simulink model "pasaBajoSimuLink"  (R2014b)
settings: Solver=ode45  StartTime=0.0  StopTime=10.0  RelTol=1e-3
settings Model: Creator=Chehin  LastModifiedBy=Chehin

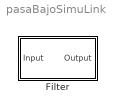
== system pasaBajoSimuLink ==
  Filter : Subsystem  Tag=FilterWizardSubSystem
      settings: ErrorFcn=dspFilterRealizedInBasicElemsAlgLoopErrFcnCallback

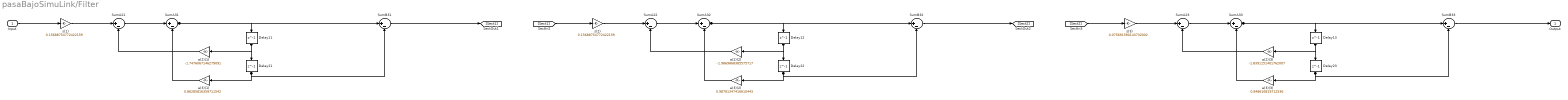
== system pasaBajoSimuLink/Filter ==
  Input : Inport
  Delay{11..13,21..23} (6 alike) : Delay  DelayLength=1  InitialCondition=0
  SumA{21..23,31..33} (6 alike) : Sum  Inputs=|+-  RndMeth=Nearest  SaturateOnIntegerOverflow=on  OutDataTypeStr=Inherit: Same as first input
  SumB31 : Sum  Inputs=|+-  RndMeth=Nearest  SaturateOnIntegerOverflow=on  OutDataTypeStr=Inherit: Same as first input
  SumB32 : Sum  Inputs=|+-  RndMeth=Nearest  SaturateOnIntegerOverflow=on  OutDataTypeStr=Inherit: Same as first input
  SumB33 : Sum  Inputs=|+-  RndMeth=Nearest  SaturateOnIntegerOverflow=on  OutDataTypeStr=Inherit: Same as first input
  a(2)(1) : Gain  Gain=-1.7476067146279091  ParamDataTypeStr=double  RndMeth=Nearest  SaturateOnIntegerOverflow=on  OutDataTypeStr=Inherit: Same as input
  a(2)(2) : Gain  Gain=-1.9869868385575717  ParamDataTypeStr=double  RndMeth=Nearest  SaturateOnIntegerOverflow=on  OutDataTypeStr=Inherit: Same as input
  a(2)(3) : Gain  Gain=-1.8391151401762007  ParamDataTypeStr=double  RndMeth=Nearest  SaturateOnIntegerOverflow=on  OutDataTypeStr=Inherit: Same as input
  a(3)(1) : Gain  Gain=0.86285816359711542  ParamDataTypeStr=double  RndMeth=Nearest  SaturateOnIntegerOverflow=on  OutDataTypeStr=Inherit: Same as input
  a(3)(2) : Gain  Gain=0.98781347416610443  ParamDataTypeStr=double  RndMeth=Nearest  SaturateOnIntegerOverflow=on  OutDataTypeStr=Inherit: Same as input
  a(3)(3) : Gain  Gain=0.848616819712536  ParamDataTypeStr=double  RndMeth=Nearest  SaturateOnIntegerOverflow=on  OutDataTypeStr=Inherit: Same as input
  s(1) : Gain  Gain=0.15688754772422159  ParamDataTypeStr=double  RndMeth=Nearest  SaturateOnIntegerOverflow=on  OutDataTypeStr=Inherit: Same as input
  s(2) : Gain  Gain=0.15688754772422159  ParamDataTypeStr=double  RndMeth=Nearest  SaturateOnIntegerOverflow=on  OutDataTypeStr=Inherit: Same as input
  s(3) : Gain  Gain=0.075691590143732002  ParamDataTypeStr=double  RndMeth=Nearest  SaturateOnIntegerOverflow=on  OutDataTypeStr=Inherit: Same as input
  Output : Outport
  wires:
  Input/1 -> s(1)/1
  s(1)/1 -> SumA21/1
  SumA21/1 -> SumA31/1
  SumA31/1 -> SumB31/1, Delay11/1
  SumB31/1 -> [Sect1]
  a(2)(1)/1 -> SumA21/2
  Delay11/1 -> a(2)(1)/1, Delay21/1
  a(3)(1)/1 -> SumA31/2
  Delay21/1 -> a(3)(1)/1, SumB31/2
  [Sect1] -> s(2)/1
  s(2)/1 -> SumA22/1
  SumA22/1 -> SumA32/1
  SumA32/1 -> SumB32/1, Delay12/1
  SumB32/1 -> [Sect2]
  a(2)(2)/1 -> SumA22/2
  Delay12/1 -> a(2)(2)/1, Delay22/1
  a(3)(2)/1 -> SumA32/2
  Delay22/1 -> a(3)(2)/1, SumB32/2
  [Sect2] -> s(3)/1
  s(3)/1 -> SumA23/1
  SumA23/1 -> SumA33/1
  SumA33/1 -> SumB33/1, Delay13/1
  SumB33/1 -> Output/1
  a(2)(3)/1 -> SumA23/2
  Delay13/1 -> a(2)(3)/1, Delay23/1
  a(3)(3)/1 -> SumA33/2
  Delay23/1 -> a(3)(3)/1, SumB33/2
